simulink model "CartPendSim"  (R2023a)
settings: Solver=ode5  StartTime=0.0  StopTime=t_end  FixedStep=Ts  RelTol=1e-3
values from neighbouring files (symbols this model uses):
  fc = 2.0991020428    [CartPendParams.mat]
  fs = 1.55542636712    [CartPendParams.mat]
  g = 9.81    [CartPendParams.mat]
  Jp = 0.00800173441225    [CartPendParams.mat]
  K = [-3.16227766017 6.83453565636 -2.2492261796 1.40001367478]    [CartPendParams.mat]
  l = 0.0191003776244    [CartPendParams.mat]
  lpo = 0.20854    [CartPendParams.mat]
  lpwo = 0.455840449763    [CartPendParams.mat]
  m = 1    [CartPendParams.mat]
  mps = 0.0417185657763    [CartPendParams.mat]
  mpw = 0.0272036144897    [CartPendParams.mat]
  p1 = 19.442829589    [CartPendParams.mat]
  p2 = -1.26371742429    [CartPendParams.mat]
undefined symbols (not defined in the file or in its folder): cartFix, t_end, Ts, x0
libraries: simulink x1, rllib x1
settings Model: Creator=student
settings OptimizationCC: ReuseModelBlockBuffer=off
settings DebuggingCC: UnconnectedInputMsg=warning  UnconnectedOutputMsg=warning  UnconnectedLineMsg=warning
settings ModelReferenceCC: EnableRefExpFcnMdlSchedulingChecks=on
settings RTWCC: DLArmComputeVersion=19.05

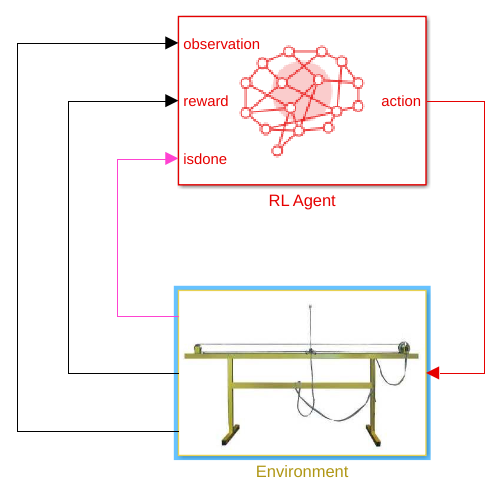
[thumbnail: Simulink's stored preview of the top-level diagram]
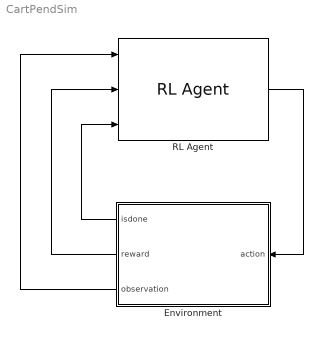
== system CartPendSim ==
  Environment : Subsystem
      mask Display: image('$imagefile'); % Use "Edit Image" on toolstrip to change.
  RL Agent : rllib/RL Agent  Agent=agent  ExternalActionAsInput=off  ProvideLastAction=off  ProvideCumRwd=off  TreatAsDirectFeedthrough=on  UseStrictObservationDataTypes=off
  wires:
  RL Agent/1 -> Environment/1(action)
  Environment/3(observation) -> RL Agent/1
  Environment/1(isdone) -> RL Agent/3
  Environment/2(reward) -> RL Agent/2

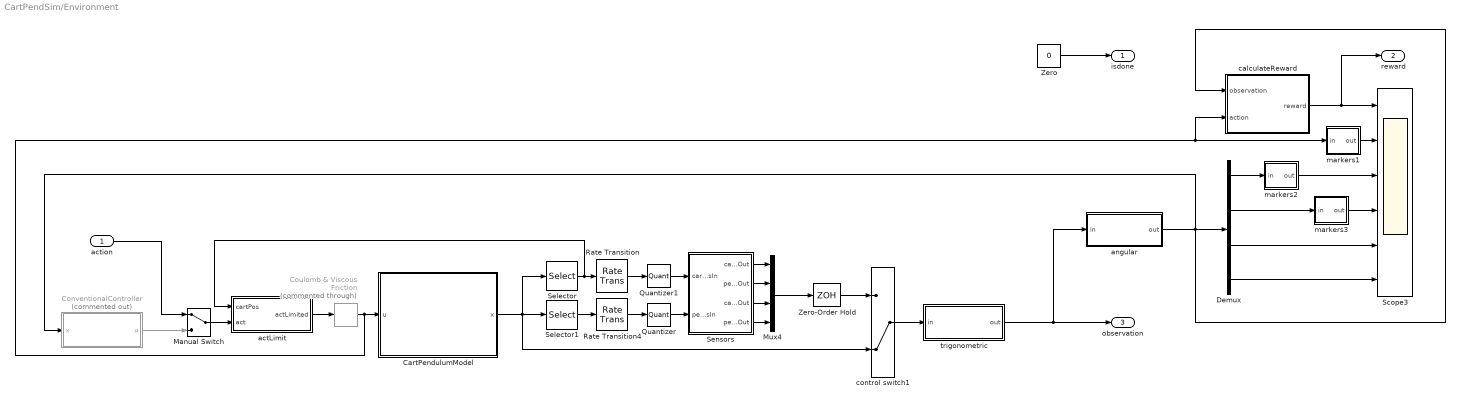
== system CartPendSim/Environment ==
  action : Inport
  CartPendulumModel : Subsystem
  ConventionalController : Subsystem  Commented=on
  Coulomb & Viscous Friction : simulink/Discontinuities/Coulomb & Viscous Friction  Commented=through  offset=0.08  gain=1
  Demux : Demux
  Manual Switch : ManualSwitch
  Mux4 : Mux
  Quantizer : Quantizer  QuantizationInterval=2*pi /4096
  Quantizer1 : Quantizer  QuantizationInterval=1 /17381
  Rate Transition : RateTransition  InitialCondition=x0(1)  OutPortSampleTime=Ts
  Rate Transition4 : RateTransition  InitialCondition=x0(2)  OutPortSampleTime=Ts
  Scope3 : Scope  NumInputPorts=6
  Selector : Selector  InputPortWidth=4  IndexOptions=Index vector (dialog)  Indices=[1]  OutputSizes=1
  Selector1 : Selector  InputPortWidth=4  IndexOptions=Index vector (dialog)  Indices=[2]  OutputSizes=1
  Sensors : Subsystem  mask(PENDULUM Output){T0=Ts}
      mask prompts: T0 "Sample Time"
      mask help: PCL-812 PG Device Driver
  Zero : Constant  Value=0  OutDataTypeStr=Inherit: Inherit via back propagation
  Zero-Order Hold : ZeroOrderHold  SampleTime=Ts
  actLimit : Subsystem
  angular : Subsystem
  calculateReward : Subsystem
  control switch1 : ManualSwitch  CurrentSetting=0
  markers1 : Subsystem
  markers2 : Subsystem
  markers3 : Subsystem
  trigonometric : Subsystem
  isdone : Outport
  reward : Outport  Port=2
  observation : Outport  Port=3
  wires:
  actLimit/1(actLimited) -> Coulomb & Viscous Friction/1
  action/1 -> Manual Switch/1
  calculateReward/1(reward) -> reward/1, Scope3/1
  Sensors/4(pendVelOut) -> Mux4/4
  Sensors/2(pendPosOut) -> Mux4/2
  Quantizer/1 -> Sensors/2(pendPosIn)
  Sensors/3(cartVelOut) -> Mux4/3
  Sensors/1(cartPosOut) -> Mux4/1
  Rate Transition4/1 -> Quantizer/1
  Rate Transition/1 -> Quantizer1/1
  Selector1/1 -> Rate Transition4/1
  Mux4/1 -> Zero-Order Hold/1
  control switch1/1 -> trigonometric/1(in)
  trigonometric/1(out) -> angular/1(in), observation/1
  Demux/4 -> Scope3/6
  Demux/3 -> Scope3/5
  Demux/2 -> markers3/1(in)
  Demux/1 -> markers2/1(in)
  Coulomb & Viscous Friction/1 -> CartPendulumModel/1(u), markers1/1(in), calculateReward/2(action)
  markers2/1(out) -> Scope3/3
  markers3/1(out) -> Scope3/4
  Quantizer1/1 -> Sensors/1(cartPosIn)
  Zero-Order Hold/1 -> control switch1/1
  CartPendulumModel/1(x) -> control switch1/2, Selector1/1, Selector/1
  Selector/1 -> actLimit/1(cartPos), Rate Transition/1
  markers1/1(out) -> Scope3/2
  Zero/1 -> isdone/1
  ConventionalController/1(u) -> Manual Switch/2
  angular/1(out) -> calculateReward/1(observation), ConventionalController/1(x), Demux/1
  Manual Switch/1 -> actLimit/2(act)

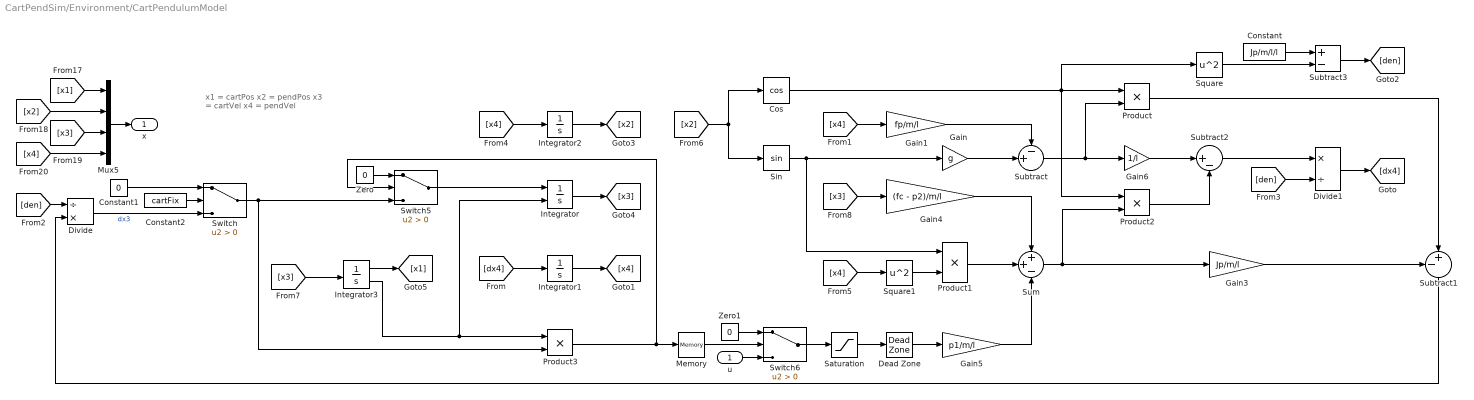
== system CartPendSim/Environment/CartPendulumModel ==
  note: x1 = cartPos
      | x2 = pendPos
      | x3 = cartVel
      | x4 = pendVel
  u : Inport
  Constant : Constant  Value=Jp/m/l/l
  Constant1 : Constant  Value=0
  Constant2 : Constant  Value=cartFix
  Cos : Trigonometry  Operator=cos
  Dead Zone : DeadZone  LowerValue=-fs/p1  UpperValue=fs/p1
  Divide : Product  Inputs=/*
  Divide1 : Product  Inputs=*/
  Gain : Gain  Gain=g
  Gain1 : Gain  Gain=fp/m/l
  Gain3 : Gain  Gain=Jp/m/l
  Gain4 : Gain  Gain=(fc - p2)/m/l
  Gain5 : Gain  Gain=p1/m/l
  Gain6 : Gain  Gain=1/l
  Integrator : Integrator  ExternalReset=either  InitialCondition=x0(3)
  Integrator1 : Integrator  InitialCondition=x0(4)
  Integrator2 : Integrator  InitialCondition=x0(2)
  Integrator3 : Integrator  InitialCondition=x0(1)  LimitOutput=on  UpperSaturationLimit=0.9  LowerSaturationLimit=-0.9  ShowSaturationPort=on
  Memory : Memory
  Mux5 : Mux
  Product{,1..3} (4 alike) : Product
  Saturation : Saturate
  Sin : Trigonometry
  Square : Math  Operator=square
  Square1 : Math  Operator=square
  Subtract : Sum  Inputs=-+|
  Subtract1 : Sum  Inputs=-+|
  Subtract2 : Sum  Inputs=|+-
  Subtract3 : Sum  Inputs=+-
  Sum : Sum  Inputs=++-
  Switch : Switch  Criteria=u2 > Threshold  SaturateOnIntegerOverflow=off  InputSameDT=off
  Switch5 : Switch  Criteria=u2 > Threshold  SaturateOnIntegerOverflow=off  InputSameDT=off
  Switch6 : Switch  Criteria=u2 > Threshold  SaturateOnIntegerOverflow=off  InputSameDT=off
  Zero : Constant  Value=0  OutDataTypeStr=Inherit: Inherit via back propagation
  Zero1 : Constant  Value=0  OutDataTypeStr=Inherit: Inherit via back propagation
  x : Outport  PortDimensions=4
  wires:
  [dx4] -> Integrator1/1
  Gain4/1 -> Sum/1
  Sum/1 -> Product2/2, Gain3/1
  Subtract2/1 -> Divide1/1
  Subtract3/1 -> [den]
  Square/1 -> Subtract3/2
  Product1/1 -> Sum/2
  [den] -> Divide/1
  Constant2/1 -> Switch/2
  Constant/1 -> Subtract3/1
  Product2/1 -> Subtract2/2
  Gain/1 -> Subtract/2
  Gain3/1 -> Subtract1/1
  Cos/1 -> Product2/1, Product/1, Square/1
  [x4] -> Gain1/1
  Subtract/1 -> Product/2, Gain6/1
  [x4] -> Integrator2/1
  Saturation/1 -> Dead Zone/1
  Gain1/1 -> Subtract/1
  Gain6/1 -> Subtract2/1
  [den] -> Divide1/2
  Product/1 -> Subtract1/2
  Divide1/1 -> [dx4]
  Divide/1 -> Switch/3  "dx3"
  Subtract1/1 -> Divide/2
  Square1/1 -> Product1/2
  Sin/1 -> Gain/1, Product1/1
  [x2] -> Sin/1, Cos/1
  Integrator3/1 -> [x1]
  Mux5/1 -> x/1
  Dead Zone/1 -> Gain5/1
  Constant1/1 -> Switch/1
  Integrator/1 -> [x3]
  [x1] -> Mux5/1
  [x2] -> Mux5/2
  [x3] -> Mux5/3
  [x4] -> Mux5/4
  Integrator3/2 -> Product3/1, Integrator/2
  Switch/1 -> Switch5/3, Product3/2
  Switch5/1 -> Integrator/1
  Zero/1 -> Switch5/1
  Zero1/1 -> Switch6/1
  Product3/1 -> Memory/1, Switch5/2
  u/1 -> Switch6/3
  Memory/1 -> Switch6/2
  Switch6/1 -> Saturation/1
  Integrator1/1 -> [x4]
  [x4] -> Square1/1
  Integrator2/1 -> [x2]
  [x3] -> Integrator3/1
  [x3] -> Gain4/1
  Gain5/1 -> Sum/3

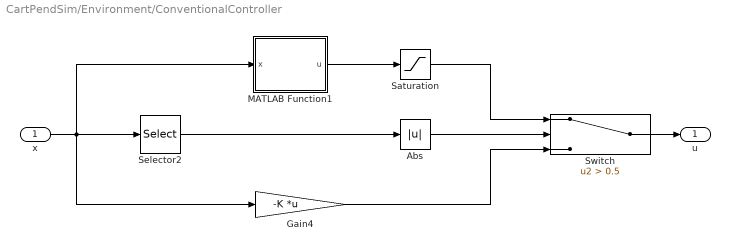
== system CartPendSim/Environment/ConventionalController ==
  x : Inport
  Abs : Abs  SaturateOnIntegerOverflow=off
  Gain4 : Gain  Gain=-K  Multiplication=Matrix(K*u) (u vector)
  MATLAB Function1 : MATLAB Function  TreatAsAtomicUnit=on
  Saturation : Saturate  UpperLimit=0.4  LowerLimit=-0.4
  Selector2 : Selector  InputPortWidth=4  IndexOptions=Index vector (dialog)  Indices=[2]  OutputSizes=1
  Switch : Switch  Criteria=u2 > Threshold  Threshold=0.5  SaturateOnIntegerOverflow=off  InputSameDT=off
  u : Outport
  wires:
  Abs/1 -> Switch/2
  MATLAB Function1/1(u) -> Saturation/1
  x/1 -> Gain4/1, Selector2/1, MATLAB Function1/1(x)
  Selector2/1 -> Abs/1
  Switch/1 -> u/1
  Saturation/1 -> Switch/1
  Gain4/1 -> Switch/3

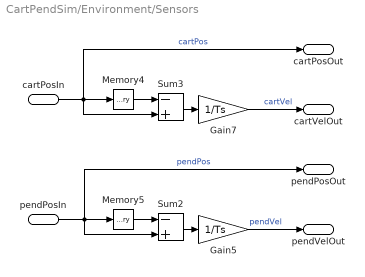
== system CartPendSim/Environment/Sensors ==
  cartPosIn : Inport
  pendPosIn : Inport  Port=2
  Gain5 : Gain  Gain=1/Ts  SaturateOnIntegerOverflow=on  OutDataTypeStr=Inherit: Same as input  ParamDataTypeStr=Inherit: Same as input
  Gain7 : Gain  Gain=1/Ts  SaturateOnIntegerOverflow=on  OutDataTypeStr=Inherit: Same as input  ParamDataTypeStr=Inherit: Same as input
  Memory4 : Memory  InitialCondition=x0(1)  InheritSampleTime=on
  Memory5 : Memory  InitialCondition=x0(2)  InheritSampleTime=on
  Sum2 : Sum  Inputs=-+  InputSameDT=on  SaturateOnIntegerOverflow=on  OutDataTypeStr=Inherit: Same as first input
  Sum3 : Sum  Inputs=-+  InputSameDT=on  SaturateOnIntegerOverflow=on  OutDataTypeStr=Inherit: Same as first input
  cartPosOut : Outport  InitialOutput=0
  pendPosOut : Outport  Port=2  InitialOutput=0
  cartVelOut : Outport  Port=3  InitialOutput=0
  pendVelOut : Outport  Port=4  InitialOutput=0
  wires:
  cartPosIn/1 -> cartPosOut/1, Memory4/1, Sum3/2  "cartPos"
  Gain5/1 -> pendVelOut/1  "pendVel"
  pendPosIn/1 -> Memory5/1, Sum2/2, pendPosOut/1  "pendPos"
  Gain7/1 -> cartVelOut/1  "cartVel"
  Sum3/1 -> Gain7/1
  Memory5/1 -> Sum2/1
  Memory4/1 -> Sum3/1
  Sum2/1 -> Gain5/1

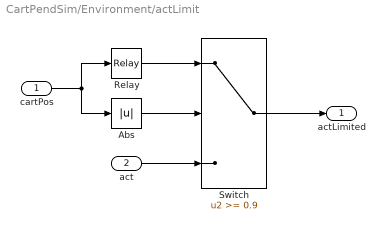
== system CartPendSim/Environment/actLimit ==
  cartPos : Inport
  act : Inport  Port=2
  Abs : Abs  SaturateOnIntegerOverflow=off
  Relay : Relay  OnSwitchValue=0  OffSwitchValue=0  OnOutputValue=-0.1  OffOutputValue=0.1
  Switch : Switch  Threshold=0.9  SaturateOnIntegerOverflow=off  InputSameDT=off
  actLimited : Outport
  wires:
  Abs/1 -> Switch/2
  act/1 -> Switch/3
  Switch/1 -> actLimited/1
  Relay/1 -> Switch/1
  cartPos/1 -> Abs/1, Relay/1

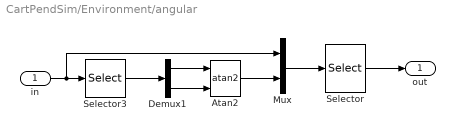
== system CartPendSim/Environment/angular ==
  in : Inport
  Atan2 : Trigonometry  Operator=atan2
  Demux1 : Demux  Outputs=2
  Mux : Mux  Inputs=2
  Selector : Selector  InputPortWidth=6  IndexOptions=Index vector (dialog)  Indices=[1 6 4 5]  OutputSizes=1
  Selector3 : Selector  InputPortWidth=5  IndexOptions=Index vector (dialog)  Indices=[2 3]  OutputSizes=1
  out : Outport
  wires:
  Demux1/1 -> Atan2/1
  Demux1/2 -> Atan2/2
  in/1 -> Mux/1, Selector3/1
  Selector3/1 -> Demux1/1
  Atan2/1 -> Mux/2
  Mux/1 -> Selector/1
  Selector/1 -> out/1

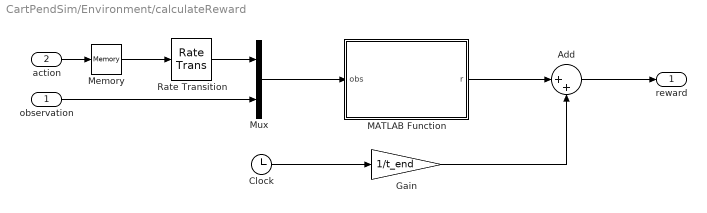
== system CartPendSim/Environment/calculateReward ==
  observation : Inport
  action : Inport  Port=2
  Add : Sum  Inputs=|++
  Clock : Clock
  Gain : Gain  Gain=1/t_end
  MATLAB Function : MATLAB Function  TreatAsAtomicUnit=on
  Memory : Memory
  Mux : Mux  Inputs=2
  Rate Transition : RateTransition
  reward : Outport
  wires:
  action/1 -> Memory/1
  Rate Transition/1 -> Mux/1
  observation/1 -> Mux/2
  Mux/1 -> MATLAB Function/1(obs)
  Clock/1 -> Gain/1
  Add/1 -> reward/1
  Gain/1 -> Add/2
  Memory/1 -> Rate Transition/1
  MATLAB Function/1(r) -> Add/1

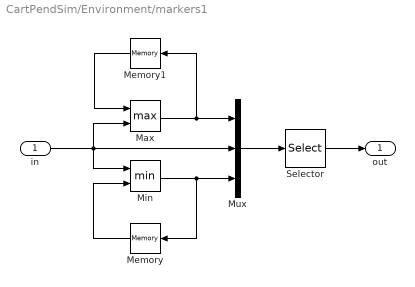
== system CartPendSim/Environment/markers1 ==
  in : Inport
  Max : MinMax  Function=max  Inputs=2
  Memory : Memory
  Memory1 : Memory
  Min : MinMax  Inputs=2
  Mux : Mux  Inputs=3
  Selector : Selector  InputPortWidth=3  IndexOptions=Index vector (dialog)  Indices=[1 3 2]  OutputSizes=1
  out : Outport
  wires:
  in/1 -> Min/1, Max/2, Mux/2
  Memory/1 -> Min/2
  Max/1 -> Mux/1, Memory1/1
  Memory1/1 -> Max/1
  Min/1 -> Mux/3, Memory/1
  Mux/1 -> Selector/1
  Selector/1 -> out/1

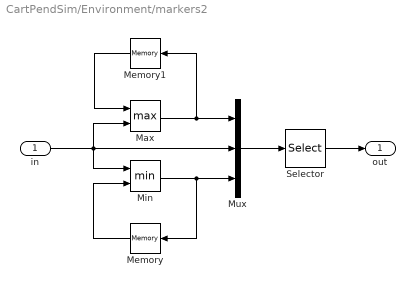
== system CartPendSim/Environment/markers2 ==
  in : Inport
  Max : MinMax  Function=max  Inputs=2
  Memory : Memory  InitialCondition=x0(1)
  Memory1 : Memory  InitialCondition=x0(1)
  Min : MinMax  Inputs=2
  Mux : Mux  Inputs=3
  Selector : Selector  InputPortWidth=3  IndexOptions=Index vector (dialog)  Indices=[1 3 2]  OutputSizes=1
  out : Outport
  wires:
  in/1 -> Min/1, Max/2, Mux/2
  Memory/1 -> Min/2
  Max/1 -> Mux/1, Memory1/1
  Memory1/1 -> Max/1
  Min/1 -> Mux/3, Memory/1
  Mux/1 -> Selector/1
  Selector/1 -> out/1

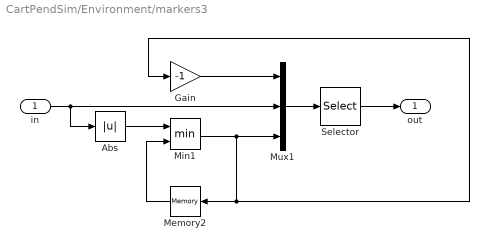
== system CartPendSim/Environment/markers3 ==
  in : Inport
  Abs : Abs  SaturateOnIntegerOverflow=off
  Gain : Gain  Gain=-1
  Memory2 : Memory  InitialCondition=x0(2)
  Min1 : MinMax  Inputs=2
  Mux1 : Mux  Inputs=3
  Selector : Selector  InputPortWidth=3  IndexOptions=Index vector (dialog)  Indices=[1 3 2]  OutputSizes=1
  out : Outport
  wires:
  in/1 -> Abs/1, Mux1/2
  Memory2/1 -> Min1/2
  Abs/1 -> Min1/1
  Mux1/1 -> Selector/1
  Gain/1 -> Mux1/1
  Min1/1 -> Memory2/1, Gain/1, Mux1/3
  Selector/1 -> out/1

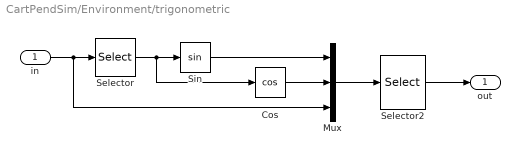
== system CartPendSim/Environment/trigonometric ==
  in : Inport
  Cos : Trigonometry  Operator=cos
  Mux : Mux  Inputs=3
  Selector : Selector  InputPortWidth=4  IndexOptions=Index vector (dialog)  Indices=2  OutputSizes=1
  Selector2 : Selector  InputPortWidth=6  IndexOptions=Index vector (dialog)  Indices=[3 1 2 5 6]  OutputSizes=1
  Sin : Trigonometry
  out : Outport
  wires:
  Sin/1 -> Mux/1
  Cos/1 -> Mux/2
  Selector/1 -> Sin/1, Cos/1
  in/1 -> Mux/3, Selector/1
  Mux/1 -> Selector2/1
  Selector2/1 -> out/1

== matlab function CartPendSim/Environment/calculateReward/MATLAB Function ==
  data: obs input; r output; mpw parameter; mps parameter; lpwo parameter; lpo parameter; g parameter; Jp parameter
function r = CalculateReward(obs, mpw, mps, lpwo, lpo, g, Jp)
    act = obs(1);
    cartPos = obs(2);
    pendPos = obs(3);
    pendVel = obs(5);

    ZeroReward = @(val) exp(-abs(val));

    r = 0;
    Ep = (mpw*lpwo + mps*lpo)*g*(cos(pendPos) + 1);
    Ek = (Jp*pendVel^2)/2;
    Em = Ep + Ek;
    Ep0 = 2*g*(mpw*lpwo + mps*lpo);

    % swing-up & balancing
    r = r + 10*ZeroReward(Em - Ep0);
    r = r + 10*(Em > Ep0)*ZeroReward(pendVel);
    r = r + 10*(sign(pendPos*cartPos) == 1);
    if (abs(pendPos) > 0.38) % swing-up
        r = r + 20*ZeroReward(10 - abs(pendVel));
    else % balancing
        r = r + 20;
        r = r + 15*ZeroReward(10*pendPos);
        r = r + 15*max(0, sign(Em - Ep0)*2*act*sign(pendPos));
        r = r + 10*ZeroReward(act);
        r = r + 10*ZeroReward(cartPos);
        r = r + 10*(sign(pendPos*pendVel) ~= 1);
    end

    if (abs(cartPos) >= 0.5 || abs(act) == 0.5)
        r = 0;
    end
end

== matlab function CartPendSim/Environment/ConventionalController/MATLAB Function1 ==
  data: x input; u output; mpw parameter; mps parameter; lpwo parameter; lpo parameter; g parameter; Jp parameter
function u = swingUp(x, mpw, mps, lpwo, lpo, g, Jp)
    pendPos = x(2);
    pendVel = x(4);
    Ep = (mpw*lpwo + mps*lpo)*g*(cos(pendPos) + 1);
    Ek = (Jp*pendVel^2)/2;
    Em = Ep + Ek;
    Ep0 = 2*g*(mpw*lpwo + mps*lpo);
    if (Em < Ep0)
        u = sign(pendVel*cos(pendPos));
    else
        u = 0;
    end
end
